simulink model "sensor"  (R2019b)
settings: Solver=VariableStepAuto  StartTime=0.0  StopTime=10.0  RelTol=1e-3
undefined symbols (not defined in the file or in its folder): sensitivity_encoder, sensitivity_giroscopio, Ts
libraries: simulink x4, dspstat3 x4, dsparch4 x2
settings Model: Creator=AndreaCalegari  LastModifiedBy=AndreaCalegari

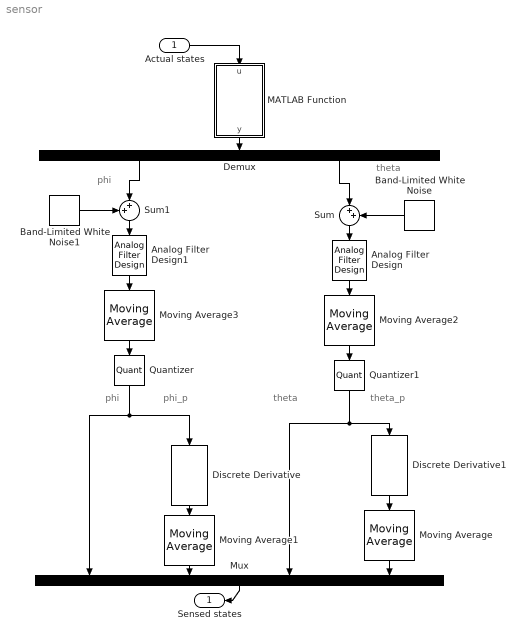
== system sensor ==
  note: theta_p
  note: phi
  note: theta
  note: phi_p
  note: phi
  note: theta
  Actual states : Inport  PortDimensions=4  SampleTime=Ts
  Analog Filter Design : dsparch4/Analog Filter Design  method=Butterworth  filttype=Lowpass  N=2  Wlo=30  Whi=80  Rp=2  Rs=40
  Analog Filter Design1 : dsparch4/Analog Filter Design  method=Butterworth  filttype=Lowpass  N=2  Wlo=30  Whi=80  Rp=2  Rs=40
  Band-Limited White Noise : simulink/Sources/Band-Limited White Noise  Cov=[0.00000001]  Ts=0.001  seed=[23341]
  Band-Limited White Noise1 : simulink/Sources/Band-Limited White Noise  Cov=[0.00000001]  Ts=0.001  seed=[23341]
  Demux : Demux  Outputs=2
  Discrete Derivative : simulink/Discrete/Discrete Derivative  gainval=1.0  ICPrevScaledInput=0.0  OutMin=[]  OutMax=[]  OutDataType=fixdt(1, 16)  OutScaling=2^-10  DoSatur=off
  Discrete Derivative1 : simulink/Discrete/Discrete Derivative  gainval=1.0  ICPrevScaledInput=0.0  OutMin=[]  OutMax=[]  OutDataType=fixdt(1, 16)  OutScaling=2^-10  DoSatur=off
  MATLAB Function : MATLAB Function  TreatAsAtomicUnit=on
  Moving Average{,1..3} (4 alike) : dspstat3/Moving Average  Method=Sliding window  ForgettingFactorPort=off  SpecifyWindowLength=on  WindowLength=200  ForgettingFactor=0.9  SimulateUsing=Code generation
  Mux : Mux
  Quantizer : Quantizer  QuantizationInterval=1/sensitivity_encoder
  Quantizer1 : Quantizer  QuantizationInterval=1/sensitivity_giroscopio
  Sum : Sum  Inputs=|++
  Sum1 : Sum  Inputs=++|
  Sensed states : Outport
  wires:
  Discrete Derivative/1 -> Moving Average1/1
  Discrete Derivative1/1 -> Moving Average/1
  Sum/1 -> Analog Filter Design/1
  Demux/2 -> Sum/1
  Sum1/1 -> Analog Filter Design1/1
  Band-Limited White Noise/1 -> Sum/2
  Quantizer1/1 -> Mux/3, Discrete Derivative1/1
  Quantizer/1 -> Mux/1, Discrete Derivative/1
  MATLAB Function/1(y) -> Demux/1
  Band-Limited White Noise1/1 -> Sum1/1
  Moving Average/1 -> Mux/4
  Demux/1 -> Sum1/2
  Mux/1 -> Sensed states/1
  Actual states/1 -> MATLAB Function/1(u)
  Moving Average1/1 -> Mux/2
  Analog Filter Design/1 -> Moving Average2/1
  Moving Average2/1 -> Quantizer1/1
  Analog Filter Design1/1 -> Moving Average3/1
  Moving Average3/1 -> Quantizer/1

== matlab function sensor/MATLAB Function ==
  data: u input; y output
function y = fcn(u)

y = [u(1),u(3)];
